simulink library "inp"  (R2021b)
settings: Solver=VariableStepAuto  StartTime=0.0  StopTime=10.0  RelTol=1e-3
undefined symbols (not defined in the file): C_TASK_5MS_S, FALSE, KINP_AcoreReadyToSlp_flg_ovrdflg, KINP_AcoreReadyToSlp_flg_ovrdval, KINP_AllowMovThd_OTA_enum_ovrdflg, KINP_AllowMovThd_OTA_enum_ovrdval, KINP_APSAngleTarget_Deg_ovrdflg, KINP_APSAngleTarget_Deg_ovrdval, KINP_APSDecReq_mps2_ovrdflg, KINP_APSDecReq_mps2_ovrdval, KINP_APSDecReqA_flg_ovrdflg, KINP_APSDecReqA_flg_ovrdval, KINP_APSDFLL_cm_ovrdflg, KINP_APSDFLL_cm_ovrdval, KINP_APSDFLR_cm_ovrdflg, KINP_APSDFLR_cm_ovrdval, KINP_APSDRLL_cm_ovrdflg, KINP_APSDRLL_cm_ovrdval, KINP_APSDRLR_cm_ovrdflg, KINP_APSDRLR_cm_ovrdval, KINP_APSExitCondition_enum_ovrdflg, KINP_APSExitCondition_enum_ovrdval, KINP_APSHWVer_enum_ovrdflg, KINP_APSHWVer_enum_ovrdval, KINP_APSProgressPCT_pct_ovrdflg, KINP_APSProgressPCT_pct_ovrdval, KINP_APSReq_enum_ovrdflg, KINP_APSReq_enum_ovrdval, KINP_APSRQDisplay_enum_ovrdflg, KINP_APSRQDisplay_enum_ovrdval, KINP_APSRqEPASCtrl_flg_ovrdflg, KINP_APSRqEPASCtrl_flg_ovrdval, KINP_APSShiftPosnReq_enum_ovrdval, KINP_APSShiftPosnReq_enum_ovrflg, KINP_APSSpeedCMD_kph_ovrdval, KINP_APSSpeedCMD_kph_ovrflg, KINP_APSStaSystem_enum_ovrdflg, KINP_APSStaSystem_enum_ovrdval, KINP_APSSWVer_enum_ovrdflg, KINP_APSSWVer_enum_ovrdval, KINP_APSVMCReqA_flg_ovrdval, KINP_APSVMCReqA_flg_ovrflg, KINP_APSVRqEPASCtrl_flg_ovrdflg, KINP_APSVRqEPASCtrl_flg_ovrdval, KINP_AuxBattVolmV_mV_ovrdflg, KINP_AuxBattVolmV_mV_ovrdval, KINP_CAASSta_enum_ovrdflg, KINP_CAASSta_enum_ovrdval, KINP_CAASVMCReqA_flg_ovrdval, KINP_CAASVMCReqA_flg_ovrflg, KINP_Chime_enum_ovrdflg, KINP_Chime_enum_ovrdval, KINP_ClearDTCcmd_flg_ovrdflg, KINP_ClearDTCcmd_flg_ovrdval, KINP_EvccAplusPwrUpReq_flg_ovrdflg, KINP_EvccAplusPwrUpReq_flg_ovrdval, KINP_LFID_raw_ovrdval, KINP_LFID_raw_ovrflg, KINP_LRID_raw_ovrdval, KINP_MemOffsetAccX_raw16_ovrdflg ... (+118)
libraries: FVT_lib x503, hcu_lib x1
(part 6 of 16)

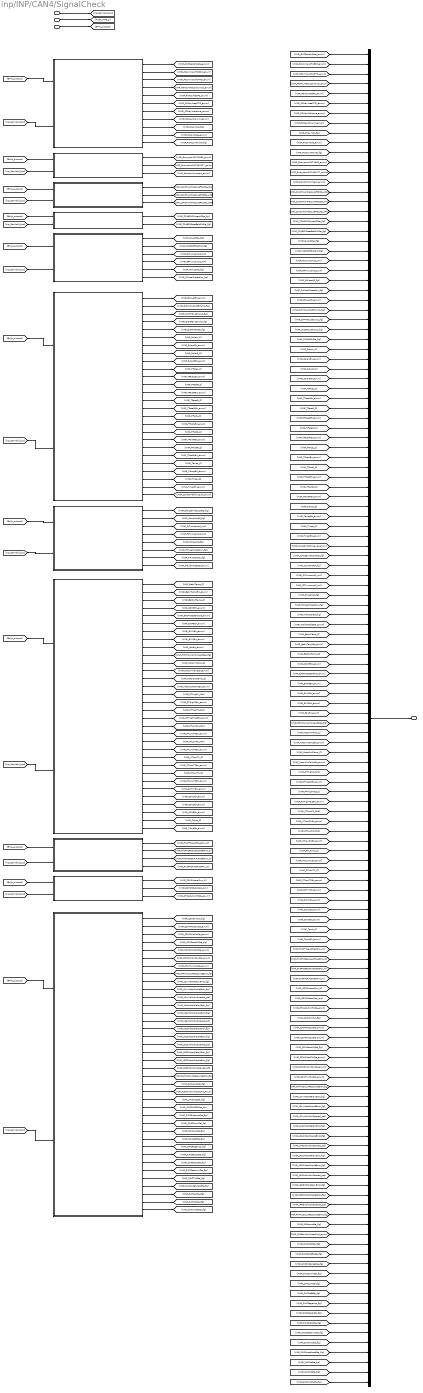
== system inp/INP/CAN4/SignalCheck ==
  inp_CanValid_bus : Inport
  TASK_TIME_S : Inport  Port=2
  BHAL_outputs : Inport  Port=3
  DKC1 : Subsystem
  DKC2 : Subsystem
  Z24_C1000_0 : Subsystem
  Z24_CE100_0 : Subsystem
  ZONE_DR1 : Subsystem
  ZONE_DR_VCU : Subsystem
  ZONE_FR1 : Subsystem
  ZONE_FR_VCU : Subsystem
  bus_creator : BusCreator  Inputs=136
  zGW_APTC1 : Subsystem
  zGW_CANFr1 : Subsystem
  zGW_LINDr1 : Subsystem
  inp_Hal_bus : Outport
  wires:
  inp_CanValid_bus/1 -> [inp_CanValid_bus]
  TASK_TIME_S/1 -> [TASK_TIME_S]
  BHAL_outputs/1 -> [BHAL_outputs]
  [BHAL_outputs] -> DKC1/1(BHAL_outputs)
  [inp_CanValid_bus] -> DKC1/2(inp_CanValid_bus)
  DKC1/1(VINP_DKCReVehData_enum) -> [VINP_DKCReVehData_enum]
  DKC1/2(VINP_PCommandToBCM_enum) -> [VINP_PCommandToBCM_enum]
  DKC1/3(VINP_PCommandToPTG_enum) -> [VINP_PCommandToPTG_enum]
  DKC1/4(VINP_PDKeyAreaLockUnlock_enum) -> [VINP_PDKeyAreaLockUnlock_enum]
  DKC1/5(VINP_PDKeyAreaPS_enum) -> [VINP_PDKeyAreaPS_enum]
  DKC1/6(VINP_PDKeyAreaPTG_enum) -> [VINP_PDKeyAreaPTG_enum]
  DKC1/7(VINP_PDKeyWelcome_enum) -> [VINP_PDKeyWelcome_enum]
  DKC1/8(VINP_PDkeyShowIVI_enum) -> [VINP_PDkeyShowIVI_enum]
  DKC1/9(VINP_PKeyMiss_flg) -> [VINP_PKeyMiss_flg]
  DKC1/10(VINP_PKeyMode_enum) -> [VINP_PKeyMode_enum]
  DKC1/11(VINP_PUIDLowPower_flg) -> [VINP_PUIDLowPower_flg]
  [BHAL_outputs] -> DKC2/1(BHAL_outputs)
  [inp_CanValid_bus] -> DKC2/2(inp_CanValid_bus)
  DKC2/1(VINP_EncryptionDATA063_enum) -> [VINP_EncryptionDATA063_enum]
  DKC2/2(VINP_EncryptionDATA64127_enum) -> [VINP_EncryptionDATA64127_enum]
  DKC2/3(VINP_RandomNumberX_enum) -> [VINP_RandomNumberX_enum]
  [BHAL_outputs] -> Z24_C1000_0/1(BHAL_outputs)
  [inp_CanValid_bus] -> Z24_C1000_0/2(inp_CanValid_bus)
  Z24_C1000_0/1(VINP_Z24CHAAirPressureFC2Sta_KPa) -> [VINP_Z24CHAAirPressureFC2Sta_KPa]
  Z24_C1000_0/2(VINP_Z24CHAAirPressurePC3Sta_KPa) -> [VINP_Z24CHAAirPressurePC3Sta_KPa]
  Z24_C1000_0/3(VINP_Z24CHAAirPressureRC1Sta_KPa) -> [VINP_Z24CHAAirPressureRC1Sta_KPa]
  [BHAL_outputs] -> Z24_CE100_0/1(BHAL_outputs)
  [inp_CanValid_bus] -> Z24_CE100_0/2(inp_CanValid_bus)
  Z24_CE100_0/1(VINP_Z24BCMFWiperASSta_flg) -> [VINP_Z24BCMFWiperASSta_flg]
  Z24_CE100_0/2(VINP_Z24BCMSeatBeltSWSta_flg) -> [VINP_Z24BCMSeatBeltSWSta_flg]
  [BHAL_outputs] -> ZONE_DR1/1(BHAL_outputs)
  [inp_CanValid_bus] -> ZONE_DR1/2(inp_CanValid_bus)
  ZONE_DR1/1(VINP_DrLockSta_flg) -> [VINP_DrLockSta_flg]
  ZONE_DR1/2(VINP_MIRRORFOLDSW_flg) -> [VINP_MIRRORFOLDSW_flg]
  ZONE_DR1/3(VINP_RLTurnLampC_mA) -> [VINP_RLTurnLampC_mA]
  ZONE_DR1/4(VINP_RRTurnLampC_mA) -> [VINP_RRTurnLampC_mA]
  ZONE_DR1/5(VINP_RWiperAS_flg) -> [VINP_RWiperAS_flg]
  ZONE_DR1/6(VINP_RWiperProtection_flg) -> [VINP_RWiperProtection_flg]
  [BHAL_outputs] -> ZONE_DR_VCU/1(BHAL_outputs)
  [inp_CanValid_bus] -> ZONE_DR_VCU/2(inp_CanValid_bus)
  ZONE_DR_VCU/1(VINP_BlowerErr_enum) -> [VINP_BlowerErr_enum]
  ZONE_DR_VCU/2(VINP_DrPMMLVOutPErrLmp_flg) -> [VINP_DrPMMLVOutPErrLmp_flg]
  ZONE_DR_VCU/3(VINP_DrPMMSysErrLmp_flg) -> [VINP_DrPMMSysErrLmp_flg]
  ZONE_DR_VCU/4(VINP_DrSCPSysErrLmp_flg) -> [VINP_DrSCPSysErrLmp_flg]
  ZONE_DR_VCU/5(VINP_DrStdAErrSta_flg) -> [VINP_DrStdAErrSta_flg]
  ZONE_DR_VCU/6(VINP_SolarL_W) -> [VINP_SolarL_W]
  ZONE_DR_VCU/7(VINP_SolarLErr_enum) -> [VINP_SolarLErr_enum]
  ZONE_DR_VCU/8(VINP_SolarR_W) -> [VINP_SolarR_W]
  ZONE_DR_VCU/9(VINP_SolarRErr_enum) -> [VINP_SolarRErr_enum]
  ZONE_DR_VCU/10(VINP_TFaceL_C) -> [VINP_TFaceL_C]
  ZONE_DR_VCU/11(VINP_TFaceLErr_enum) -> [VINP_TFaceLErr_enum]
  ZONE_DR_VCU/12(VINP_TFaceR_C) -> [VINP_TFaceR_C]
  ZONE_DR_VCU/13(VINP_TFaceRErr_enum) -> [VINP_TFaceRErr_enum]
  ZONE_DR_VCU/14(VINP_TFaceRr_C) -> [VINP_TFaceRr_C]
  ZONE_DR_VCU/15(VINP_TFaceRrErr_enum) -> [VINP_TFaceRrErr_enum]
  ZONE_DR_VCU/16(VINP_TFootL_C) -> [VINP_TFootL_C]
  ZONE_DR_VCU/17(VINP_TFootLErr_enum) -> [VINP_TFootLErr_enum]
  ZONE_DR_VCU/18(VINP_TFootR_C) -> [VINP_TFootR_C]
  ZONE_DR_VCU/19(VINP_TFootRErr_enum) -> [VINP_TFootRErr_enum]
  ZONE_DR_VCU/20(VINP_TFootRr_C) -> [VINP_TFootRr_C]
  ZONE_DR_VCU/21(VINP_TFootRrErr_enum) -> [VINP_TFootRrErr_enum]
  ZONE_DR_VCU/22(VINP_Tevap_C) -> [VINP_Tevap_C]
  ZONE_DR_VCU/23(VINP_TevapErr_enum) -> [VINP_TevapErr_enum]
  ZONE_DR_VCU/24(VINP_Tincar_C) -> [VINP_Tincar_C]
  ZONE_DR_VCU/25(VINP_TincarErr_enum) -> [VINP_TincarErr_enum]
  ZONE_DR_VCU/26(VINP_ZoneDrMalfunLevel_enum) -> [VINP_ZoneDrMalfunLevel_enum]
  [BHAL_outputs] -> ZONE_FR1/1(BHAL_outputs)
  [inp_CanValid_bus] -> ZONE_FR1/2(inp_CanValid_bus)
  ZONE_FR1/1(VINP_ChargeInletLockSta_flg) -> [VINP_ChargeInletLockSta_flg]
  ZONE_FR1/2(VINP_CompProEN_flg) -> [VINP_CompProEN_flg]
  ZONE_FR1/3(VINP_FLTurnLampC_mA) -> [VINP_FLTurnLampC_mA]
  ZONE_FR1/4(VINP_FRTurnLampC_mA) -> [VINP_FRTurnLampC_mA]
  ZONE_FR1/5(VINP_FWiperAS_flg) -> [VINP_FWiperAS_flg]
  ZONE_FR1/6(VINP_FWiperProtection_flg) -> [VINP_FWiperProtection_flg]
  ZONE_FR1/7(VINP_TrailerCheck_flg) -> [VINP_TrailerCheck_flg]
  ZONE_FR1/8(VINP_TrailerModeSta_enum) -> [VINP_TrailerModeSta_enum]
  [BHAL_outputs] -> ZONE_FR_VCU/1(BHAL_outputs)
  [inp_CanValid_bus] -> ZONE_FR_VCU/2(inp_CanValid_bus)
  ZONE_FR_VCU/1(VINP_BatInTemp_C) -> [VINP_BatInTemp_C]
  ZONE_FR_VCU/2(VINP_BatInTempErr_enum) -> [VINP_BatInTempErr_enum]
  ZONE_FR_VCU/3(VINP_BatOutTemp_C) -> [VINP_BatOutTemp_C]
  ZONE_FR_VCU/4(VINP_COMPErr_enum) -> [VINP_COMPErr_enum]
  ZONE_FR_VCU/5(VINP_EACProtectEnable_enum) -> [VINP_EACProtectEnable_enum]
  ZONE_FR_VCU/6(VINP_EWP3Err_enum) -> [VINP_EWP3Err_enum]
  ZONE_FR_VCU/7(VINP_EXV1Err_enum) -> [VINP_EXV1Err_enum]
  ZONE_FR_VCU/8(VINP_EXV2Err_enum) -> [VINP_EXV2Err_enum]
  ZONE_FR_VCU/9(VINP_FanErr_enum) -> [VINP_FanErr_enum]
  ZONE_FR_VCU/10(VINP_FrPMMLimpHomeActReq_flg) -> [VINP_FrPMMLimpHomeActReq_flg]
  ZONE_FR_VCU/11(VINP_MotorInTemp_C) -> [VINP_MotorInTemp_C]
  ZONE_FR_VCU/12(VINP_MotorInTempErr_enum) -> [VINP_MotorInTempErr_enum]
  ZONE_FR_VCU/13(VINP_MotorOutTemp_C) -> [VINP_MotorOutTemp_C]
  ZONE_FR_VCU/14(VINP_MotorOutTempErr_enum) -> [VINP_MotorOutTempErr_enum]
  ZONE_FR_VCU/15(VINP_PTHighP_KPa) -> [VINP_PTHighP_KPa]
  ZONE_FR_VCU/16(VINP_PTHighPErr_enum) -> [VINP_PTHighPErr_enum]
  ZONE_FR_VCU/17(VINP_PTHighTact_C) -> [VINP_PTHighTact_C]
  ZONE_FR_VCU/18(VINP_PTHighTactErr_enum) -> [VINP_PTHighTactErr_enum]
  ZONE_FR_VCU/19(VINP_PTLowP1_KPa) -> [VINP_PTLowP1_KPa]
  ZONE_FR_VCU/20(VINP_PTLowP1Err_enum) -> [VINP_PTLowP1Err_enum]
  ZONE_FR_VCU/21(VINP_PTLowP2_KPa) -> [VINP_PTLowP2_KPa]
  ZONE_FR_VCU/22(VINP_PTLowP2Err_enum) -> [VINP_PTLowP2Err_enum]
  ZONE_FR_VCU/23(VINP_PTLowT1_C) -> [VINP_PTLowT1_C]
  ZONE_FR_VCU/24(VINP_PTLowT1Err_enum) -> [VINP_PTLowT1Err_enum]
  ZONE_FR_VCU/25(VINP_PTLowT2_C) -> [VINP_PTLowT2_C]
  ZONE_FR_VCU/26(VINP_PTLowT2Err_enum) -> [VINP_PTLowT2Err_enum]
  ZONE_FR_VCU/27(VINP_SOTXVErr_enum) -> [VINP_SOTXVErr_enum]
  ZONE_FR_VCU/28(VINP_SOV1Err_enum) -> [VINP_SOV1Err_enum]
  ZONE_FR_VCU/29(VINP_SOV2Err_enum) -> [VINP_SOV2Err_enum]
  ZONE_FR_VCU/30(VINP_SOV3Err_enum) -> [VINP_SOV3Err_enum]
  ZONE_FR_VCU/31(VINP_Tamb_C) -> [VINP_Tamb_C]
  ZONE_FR_VCU/32(VINP_TambErr_enum) -> [VINP_TambErr_enum]
  [BHAL_outputs] -> zGW_APTC1/1(BHAL_outputs)
  [inp_CanValid_bus] -> zGW_APTC1/2(inp_CanValid_bus)
  zGW_APTC1/1(VINP_FrntPTCLeActHeatPwr_W) -> [VINP_FrntPTCLeActHeatPwr_W]
  zGW_APTC1/2(VINP_FrntPTCRearLeActHeatPwr_W) -> [VINP_FrntPTCRearLeActHeatPwr_W]
  zGW_APTC1/3(VINP_FrntPTCRearRiActHeatPwr_W) -> [VINP_FrntPTCRearRiActHeatPwr_W]
  zGW_APTC1/4(VINP_FrntPTCRiActHeatPwr_W) -> [VINP_FrntPTCRiActHeatPwr_W]
  [BHAL_outputs] -> zGW_CANFr1/1(BHAL_outputs)
  [inp_CanValid_bus] -> zGW_CANFr1/2(inp_CanValid_bus)
  zGW_CANFr1/1(VINP_COMPActualPwr_W) -> [VINP_COMPActualPwr_W]
  zGW_CANFr1/2(VINP_COMPStatorSpd_rpm) -> [VINP_COMPStatorSpd_rpm]
  zGW_CANFr1/3(VINP_PTCActuPwrHSC6_enum) -> [VINP_PTCActuPwrHSC6_enum]
  [BHAL_outputs] -> zGW_LINDr1/1(BHAL_outputs)
  [inp_CanValid_bus] -> zGW_LINDr1/2(inp_CanValid_bus)
  zGW_LINDr1/1(VINP_CSWDimSw_flg) -> [VINP_CSWDimSw_flg]
  zGW_LINDr1/2(VINP_CSWFWasSwSta_enum) -> [VINP_CSWFWasSwSta_enum]
  zGW_LINDr1/3(VINP_CSWFWipSwSta_enum) -> [VINP_CSWFWipSwSta_enum]
  zGW_LINDr1/4(VINP_CSWPassSWSta_flg) -> [VINP_CSWPassSWSta_flg]
  zGW_LINDr1/5(VINP_CSWRWasSWSta_enum) -> [VINP_CSWRWasSWSta_enum]
  zGW_LINDr1/6(VINP_CSWRWipIntSwSta_enum) -> [VINP_CSWRWipIntSwSta_enum]
  zGW_LINDr1/7(VINP_CSWTurnSwSta_enum) -> [VINP_CSWTurnSwSta_enum]
  zGW_LINDr1/8(VINP_FAPWL01LINResponseError_flg) -> [VINP_FAPWL01LINResponseError_flg]
  zGW_LINDr1/9(VINP_LDrvMotorRelayError_flg) -> [VINP_LDrvMotorRelayError_flg]
  zGW_LINDr1/10(VINP_LDrvMotorRippleError_flg) -> [VINP_LDrvMotorRippleError_flg]
  zGW_LINDr1/11(VINP_LDrvValWdwOpened_pct) -> [VINP_LDrvValWdwOpened_pct]
  zGW_LINDr1/12(VINP_LPasMotorRelayError_flg) -> [VINP_LPasMotorRelayError_flg]
  zGW_LINDr1/13(VINP_LPasMotorRippleError_flg) -> [VINP_LPasMotorRippleError_flg]
  zGW_LINDr1/14(VINP_LPasValWdwOpened_pct) -> [VINP_LPasValWdwOpened_pct]
  zGW_LINDr1/15(VINP_LRLDMotorRelayError_flg) -> [VINP_LRLDMotorRelayError_flg]
  zGW_LINDr1/16(VINP_LRLDMotorRippleError_flg) -> [VINP_LRLDMotorRippleError_flg]
  zGW_LINDr1/17(VINP_LRLDValWdwOpened_pct) -> [VINP_LRLDValWdwOpened_pct]
  zGW_LINDr1/18(VINP_LRRDMotorRelayError_flg) -> [VINP_LRRDMotorRelayError_flg]
  zGW_LINDr1/19(VINP_LRRDMotorRippleError_flg) -> [VINP_LRRDMotorRippleError_flg]
  zGW_LINDr1/20(VINP_LRRDValWdwOpened_pct) -> [VINP_LRRDValWdwOpened_pct]
  zGW_LINDr1/21(VINP_RAPWL01LINResponseError_flg) -> [VINP_RAPWL01LINResponseError_flg]
  zGW_LINDr1/22(VINP_RLSLampSta_flg) -> [VINP_RLSLampSta_flg]
  zGW_LINDr1/23(VINP_RLSRainSnrWiperCmd_enum) -> [VINP_RLSRainSnrWiperCmd_enum]
  zGW_LINDr1/24(VINP_SWCACCSta_flg) -> [VINP_SWCACCSta_flg]
  zGW_LINDr1/25(VINP_SWCCANCELSta_flg) -> [VINP_SWCCANCELSta_flg]
  zGW_LINDr1/26(VINP_SWCDistanceSta_flg) -> [VINP_SWCDistanceSta_flg]
  zGW_LINDr1/27(VINP_SWCDownSta_flg) -> [VINP_SWCDownSta_flg]
  zGW_LINDr1/28(VINP_SWCLKASta_flg) -> [VINP_SWCLKASta_flg]
  zGW_LINDr1/29(VINP_SWCLeftSta_flg) -> [VINP_SWCLeftSta_flg]
  zGW_LINDr1/30(VINP_SWCRegenUp_flg) -> [VINP_SWCRegenUp_flg]
  zGW_LINDr1/31(VINP_SWCResUpSta_flg) -> [VINP_SWCResUpSta_flg]
  zGW_LINDr1/32(VINP_SWCRightSta_flg) -> [VINP_SWCRightSta_flg]
  zGW_LINDr1/33(VINP_SWCSetdownSta_flg) -> [VINP_SWCSetdownSta_flg]
  zGW_LINDr1/34(VINP_SWCTripSta_flg) -> [VINP_SWCTripSta_flg]
  zGW_LINDr1/35(VINP_SWCUndefinedSta_flg) -> [VINP_SWCUndefinedSta_flg]
  zGW_LINDr1/36(VINP_SWCUpSta_flg) -> [VINP_SWCUpSta_flg]
  zGW_LINDr1/37(VINP_SWCVRSta_flg) -> [VINP_SWCVRSta_flg]
  zGW_LINDr1/38(VINP_SWCmodeSta_flg) -> [VINP_SWCmodeSta_flg]
  bus_creator/1 -> inp_Hal_bus/1
  [VINP_DKCReVehData_enum] -> bus_creator/1
  [VINP_PCommandToBCM_enum] -> bus_creator/2
  [VINP_PCommandToPTG_enum] -> bus_creator/3
  [VINP_PDKeyAreaLockUnlock_enum] -> bus_creator/4
  [VINP_PDKeyAreaPS_enum] -> bus_creator/5
  [VINP_PDKeyAreaPTG_enum] -> bus_creator/6
  [VINP_PDKeyWelcome_enum] -> bus_creator/7
  [VINP_PDkeyShowIVI_enum] -> bus_creator/8
  [VINP_PKeyMiss_flg] -> bus_creator/9
  [VINP_PKeyMode_enum] -> bus_creator/10
  [VINP_PUIDLowPower_flg] -> bus_creator/11
  [VINP_EncryptionDATA063_enum] -> bus_creator/12
  [VINP_EncryptionDATA64127_enum] -> bus_creator/13
  [VINP_RandomNumberX_enum] -> bus_creator/14
  [VINP_Z24CHAAirPressureFC2Sta_KPa] -> bus_creator/15
  [VINP_Z24CHAAirPressurePC3Sta_KPa] -> bus_creator/16
  [VINP_Z24CHAAirPressureRC1Sta_KPa] -> bus_creator/17
  [VINP_Z24BCMFWiperASSta_flg] -> bus_creator/18
  [VINP_Z24BCMSeatBeltSWSta_flg] -> bus_creator/19
  [VINP_DrLockSta_flg] -> bus_creator/20
  [VINP_MIRRORFOLDSW_flg] -> bus_creator/21
  [VINP_RLTurnLampC_mA] -> bus_creator/22
  [VINP_RRTurnLampC_mA] -> bus_creator/23
  [VINP_RWiperAS_flg] -> bus_creator/24
  [VINP_RWiperProtection_flg] -> bus_creator/25
  [VINP_BlowerErr_enum] -> bus_creator/26
  [VINP_DrPMMLVOutPErrLmp_flg] -> bus_creator/27
  [VINP_DrPMMSysErrLmp_flg] -> bus_creator/28
  [VINP_DrSCPSysErrLmp_flg] -> bus_creator/29
  [VINP_DrStdAErrSta_flg] -> bus_creator/30
  [VINP_SolarL_W] -> bus_creator/31
  [VINP_SolarLErr_enum] -> bus_creator/32
  [VINP_SolarR_W] -> bus_creator/33
  [VINP_SolarRErr_enum] -> bus_creator/34
  [VINP_TFaceL_C] -> bus_creator/35
  [VINP_TFaceLErr_enum] -> bus_creator/36
  [VINP_TFaceR_C] -> bus_creator/37
  [VINP_TFaceRErr_enum] -> bus_creator/38
  [VINP_TFaceRr_C] -> bus_creator/39
  [VINP_TFaceRrErr_enum] -> bus_creator/40
  [VINP_TFootL_C] -> bus_creator/41
  [VINP_TFootLErr_enum] -> bus_creator/42
  [VINP_TFootR_C] -> bus_creator/43
  [VINP_TFootRErr_enum] -> bus_creator/44
  [VINP_TFootRr_C] -> bus_creator/45
  [VINP_TFootRrErr_enum] -> bus_creator/46
  [VINP_Tevap_C] -> bus_creator/47
  [VINP_TevapErr_enum] -> bus_creator/48
  [VINP_Tincar_C] -> bus_creator/49
  [VINP_TincarErr_enum] -> bus_creator/50
  [VINP_ZoneDrMalfunLevel_enum] -> bus_creator/51
  [VINP_ChargeInletLockSta_flg] -> bus_creator/52
  [VINP_CompProEN_flg] -> bus_creator/53
  [VINP_FLTurnLampC_mA] -> bus_creator/54
  [VINP_FRTurnLampC_mA] -> bus_creator/55
  [VINP_FWiperAS_flg] -> bus_creator/56
  [VINP_FWiperProtection_flg] -> bus_creator/57
  [VINP_TrailerCheck_flg] -> bus_creator/58
  [VINP_TrailerModeSta_enum] -> bus_creator/59
  [VINP_BatInTemp_C] -> bus_creator/60
  [VINP_BatInTempErr_enum] -> bus_creator/61
  [VINP_BatOutTemp_C] -> bus_creator/62
  [VINP_COMPErr_enum] -> bus_creator/63
  [VINP_EACProtectEnable_enum] -> bus_creator/64
  [VINP_EWP3Err_enum] -> bus_creator/65
  [VINP_EXV1Err_enum] -> bus_creator/66
  [VINP_EXV2Err_enum] -> bus_creator/67
  [VINP_FanErr_enum] -> bus_creator/68
  [VINP_FrPMMLimpHomeActReq_flg] -> bus_creator/69
  [VINP_MotorInTemp_C] -> bus_creator/70
  [VINP_MotorInTempErr_enum] -> bus_creator/71
  [VINP_MotorOutTemp_C] -> bus_creator/72
  [VINP_MotorOutTempErr_enum] -> bus_creator/73
  [VINP_PTHighP_KPa] -> bus_creator/74
  [VINP_PTHighPErr_enum] -> bus_creator/75
  [VINP_PTHighTact_C] -> bus_creator/76
  [VINP_PTHighTactErr_enum] -> bus_creator/77
  [VINP_PTLowP1_KPa] -> bus_creator/78
  [VINP_PTLowP1Err_enum] -> bus_creator/79
  [VINP_PTLowP2_KPa] -> bus_creator/80
  [VINP_PTLowP2Err_enum] -> bus_creator/81
  [VINP_PTLowT1_C] -> bus_creator/82
  [VINP_PTLowT1Err_enum] -> bus_creator/83
  [VINP_PTLowT2_C] -> bus_creator/84
  [VINP_PTLowT2Err_enum] -> bus_creator/85
  [VINP_SOTXVErr_enum] -> bus_creator/86
  [VINP_SOV1Err_enum] -> bus_creator/87
  [VINP_SOV2Err_enum] -> bus_creator/88
  [VINP_SOV3Err_enum] -> bus_creator/89
  [VINP_Tamb_C] -> bus_creator/90
  [VINP_TambErr_enum] -> bus_creator/91
  [VINP_FrntPTCLeActHeatPwr_W] -> bus_creator/92
  [VINP_FrntPTCRearLeActHeatPwr_W] -> bus_creator/93
  [VINP_FrntPTCRearRiActHeatPwr_W] -> bus_creator/94
  [VINP_FrntPTCRiActHeatPwr_W] -> bus_creator/95
  [VINP_COMPActualPwr_W] -> bus_creator/96
  [VINP_COMPStatorSpd_rpm] -> bus_creator/97
  [VINP_PTCActuPwrHSC6_enum] -> bus_creator/98
  [VINP_CSWDimSw_flg] -> bus_creator/99
  [VINP_CSWFWasSwSta_enum] -> bus_creator/100
  [VINP_CSWFWipSwSta_enum] -> bus_creator/101
  [VINP_CSWPassSWSta_flg] -> bus_creator/102
  [VINP_CSWRWasSWSta_enum] -> bus_creator/103
  [VINP_CSWRWipIntSwSta_enum] -> bus_creator/104
  [VINP_CSWTurnSwSta_enum] -> bus_creator/105
  [VINP_FAPWL01LINResponseError_flg] -> bus_creator/106
  [VINP_LDrvMotorRelayError_flg] -> bus_creator/107
  [VINP_LDrvMotorRippleError_flg] -> bus_creator/108
  [VINP_LDrvValWdwOpened_pct] -> bus_creator/109
  [VINP_LPasMotorRelayError_flg] -> bus_creator/110
  [VINP_LPasMotorRippleError_flg] -> bus_creator/111
  [VINP_LPasValWdwOpened_pct] -> bus_creator/112
  [VINP_LRLDMotorRelayError_flg] -> bus_creator/113
  [VINP_LRLDMotorRippleError_flg] -> bus_creator/114
  [VINP_LRLDValWdwOpened_pct] -> bus_creator/115
  [VINP_LRRDMotorRelayError_flg] -> bus_creator/116
  [VINP_LRRDMotorRippleError_flg] -> bus_creator/117
  [VINP_LRRDValWdwOpened_pct] -> bus_creator/118
  [VINP_RAPWL01LINResponseError_flg] -> bus_creator/119
  [VINP_RLSLampSta_flg] -> bus_creator/120
  [VINP_RLSRainSnrWiperCmd_enum] -> bus_creator/121
  [VINP_SWCACCSta_flg] -> bus_creator/122
  [VINP_SWCCANCELSta_flg] -> bus_creator/123
  [VINP_SWCDistanceSta_flg] -> bus_creator/124
  [VINP_SWCDownSta_flg] -> bus_creator/125
  [VINP_SWCLKASta_flg] -> bus_creator/126
  [VINP_SWCLeftSta_flg] -> bus_creator/127
  [VINP_SWCRegenUp_flg] -> bus_creator/128
  [VINP_SWCResUpSta_flg] -> bus_creator/129
  [VINP_SWCRightSta_flg] -> bus_creator/130
  [VINP_SWCSetdownSta_flg] -> bus_creator/131
  [VINP_SWCTripSta_flg] -> bus_creator/132
  [VINP_SWCUndefinedSta_flg] -> bus_creator/133
  [VINP_SWCUpSta_flg] -> bus_creator/134
  [VINP_SWCVRSta_flg] -> bus_creator/135
  [VINP_SWCmodeSta_flg] -> bus_creator/136

== system inp/INP/CAN5/CommunicationCheck ==
  BHAL_outputs : Inport
  CANMsgInvalidTBOX1 : FVT_lib/inp/CAN_Msg_Validity_Process_template  SystemSampleTime=-1  VariantActivationTime=update diagram  Latency=0  AutoFrameSizeCalculation=off
      link override ovrdflg: Value=KINP_CANMsgInvalidTBOX1_flg_ovrdflg
      link override ovrdval: Value=KINP_CANMsgInvalidTBOX1_flg_ovrdval
  CANMsgInvalidTBOX2 : FVT_lib/inp/CAN_Msg_Validity_Process_template  SystemSampleTime=-1  VariantActivationTime=update diagram  Latency=0  AutoFrameSizeCalculation=off
      link override ovrdflg: Value=KINP_CANMsgInvalidTBOX2_flg_ovrdflg
      link override ovrdval: Value=KINP_CANMsgInvalidTBOX2_flg_ovrdval
  CANMsgInvalidTBOX3 : FVT_lib/inp/CAN_Msg_Validity_Process_template  SystemSampleTime=-1  VariantActivationTime=update diagram  Latency=0  AutoFrameSizeCalculation=off
      link override ovrdflg: Value=KINP_CANMsgInvalidTBOX3_flg_ovrdflg
      link override ovrdval: Value=KINP_CANMsgInvalidTBOX3_flg_ovrdval
  bus_creator : BusCreator  Inputs=3
  bus_selector : BusSelector  OutputSignals=VHAL_CANMsgInvalidTBOX1_flg,VHAL_CANMsgInvalidTBOX2_flg,VHAL_CANMsgInvalidTBOX3_flg
  not1 : Logic  Operator=NOT  AllPortsSameDT=off  OutDataTypeStr=boolean
  not2 : Logic  Operator=NOT  AllPortsSameDT=off  OutDataTypeStr=boolean
  not3 : Logic  Operator=NOT  AllPortsSameDT=off  OutDataTypeStr=boolean
  inp_CanValid_bus : Outport
  wires:
  BHAL_outputs/1 -> [BHAL_outputs]
  bus_selector/1 -> CANMsgInvalidTBOX1/1  "<VHAL_CANMsgInvalidTBOX1_flg>"
  CANMsgInvalidTBOX1/1 -> not1/1
  not1/1 -> bus_creator/1  "VINP_CANMsgValidTBOX1_flg"
  bus_selector/2 -> CANMsgInvalidTBOX2/1  "<VHAL_CANMsgInvalidTBOX2_flg>"
  CANMsgInvalidTBOX2/1 -> not2/1
  not2/1 -> bus_creator/2  "VINP_CANMsgValidTBOX2_flg"
  bus_selector/3 -> CANMsgInvalidTBOX3/1  "<VHAL_CANMsgInvalidTBOX3_flg>"
  CANMsgInvalidTBOX3/1 -> not3/1
  not3/1 -> bus_creator/3  "VINP_CANMsgValidTBOX3_flg"
  [BHAL_outputs] -> bus_selector/1
  bus_creator/1 -> inp_CanValid_bus/1

== system inp/INP/CAN5/CreateBus ==
  inp_CanValid_bus : Inport
  inp_Hal_bus : Inport  Port=2
  UnitConverter_{1..3,9,11} (5 alike) : DataTypeConversion  OutDataTypeStr=boolean
  UnitConverter_{5,10,14..30} (19 alike) : DataTypeConversion  OutDataTypeStr=single
  UnitConverter_{4,6,8,12..13} (5 alike) : DataTypeConversion  OutDataTypeStr=uint8
  UnitConverter_31 : DataTypeConversion  OutDataTypeStr=uint32
  UnitConverter_32 : DataTypeConversion  OutDataTypeStr=uint32
  UnitConverter_7 : DataTypeConversion  OutDataTypeStr=uint16
  bus_creator : BusCreator  Inputs=32
  bus_selector : BusSelector  OutputSignals=VINP_CANMsgValidTBOX1_flg,VINP_CANMsgValidTBOX2_flg,VINP_CANMsgValidTBOX3_flg
  bus_selector_1 : BusSelector  OutputSignals=VINP_CbnPreACEnaReq_enum,VINP_PowerOffTSet_cnt,VINP_ReOutsideMirror_enum,VINP_ReDoorLock_enum,VINP_RePwrReqTbox_enum,VINP_ReRadio_flg,VINP_RemoteACTemp_C,VINP_RemoteAutoReq_flg,VINP_TBOXNETSIGSTR_enum,VINP_TBOXTESTSTATUS_enum,VINP_TimeSyncFromBSDay_DAY,VINP_TimeSyncFromBSHour_hr,VINP_TimeSyncFromBSMinute_min,VINP_TimeSyncFromBSMonth_MONTH,VINP_TimeSyncFromBSSecond_s,VINP_TimeSyncFromBSYear_YEAR,VINP_ChargePercentSet_pct,VINP_ReserveChargeOFFDay_DAY,VINP_ReserveChargeOFFHour_hr,VINP_ReserveChargeOFFMinute_min,VINP_ReserveChargeOFFMonth_MONTH,VINP_ReserveChargeOFFYear_YEAR,VINP_ReserveChargeOnDay_DAY,VINP_ReserveChargeOnHour_hr,VINP_ReserveChargeOnMinute_min,VINP_ReserveChargeOnMonth_MONTH,VINP_ReserveChargeOnYear_YEAR,VINP_TBOXHWVER_enum,VINP_TBOXSWVER_enum
  BINP_outputs : Outport
  wires:
  inp_CanValid_bus/1 -> [inp_CanValid_bus]
  inp_Hal_bus/1 -> [inp_Hal_bus]
  bus_selector/1 -> UnitConverter_1/1  "<VINP_CANMsgValidTBOX1_flg>"
  UnitConverter_1/1 -> bus_creator/1  "VINP_CANMsgValidTBOX1_flg"
  bus_selector/2 -> UnitConverter_2/1  "<VINP_CANMsgValidTBOX2_flg>"
  UnitConverter_2/1 -> bus_creator/2  "VINP_CANMsgValidTBOX2_flg"
  bus_selector/3 -> UnitConverter_3/1  "<VINP_CANMsgValidTBOX3_flg>"
  UnitConverter_3/1 -> bus_creator/3  "VINP_CANMsgValidTBOX3_flg"
  bus_selector_1/1 -> UnitConverter_4/1  "<VINP_CbnPreACEnaReq_enum>"
  UnitConverter_4/1 -> bus_creator/4  "VINP_CbnPreACEnaReq_enum"
  bus_selector_1/2 -> UnitConverter_5/1  "<VINP_PowerOffTSet_cnt>"
  UnitConverter_5/1 -> bus_creator/5  "VINP_PowerOffTSet_cnt"
  bus_selector_1/3 -> UnitConverter_6/1  "<VINP_ReOutsideMirror_enum>"
  UnitConverter_6/1 -> bus_creator/6  "VINP_ReOutsideMirror_enum"
  bus_selector_1/4 -> UnitConverter_7/1  "<VINP_ReDoorLock_enum>"
  UnitConverter_7/1 -> bus_creator/7  "VINP_ReDoorLock_enum"
  bus_selector_1/5 -> UnitConverter_8/1  "<VINP_RePwrReqTbox_enum>"
  UnitConverter_8/1 -> bus_creator/8  "VINP_RePwrReqTbox_enum"
  bus_selector_1/6 -> UnitConverter_9/1  "<VINP_ReRadio_flg>"
  UnitConverter_9/1 -> bus_creator/9  "VINP_ReRadio_flg"
  bus_selector_1/7 -> UnitConverter_10/1  "<VINP_RemoteACTemp_C>"
  UnitConverter_10/1 -> bus_creator/10  "VINP_RemoteACTemp_C"
  bus_selector_1/8 -> UnitConverter_11/1  "<VINP_RemoteAutoReq_flg>"
  UnitConverter_11/1 -> bus_creator/11  "VINP_RemoteAutoReq_flg"
  bus_selector_1/9 -> UnitConverter_12/1  "<VINP_TBOXNETSIGSTR_enum>"
  UnitConverter_12/1 -> bus_creator/12  "VINP_TBOXNETSIGSTR_enum"
  bus_selector_1/10 -> UnitConverter_13/1  "<VINP_TBOXTESTSTATUS_enum>"
  UnitConverter_13/1 -> bus_creator/13  "VINP_TBOXTESTSTATUS_enum"
  bus_selector_1/11 -> UnitConverter_14/1  "<VINP_TimeSyncFromBSDay_DAY>"
  UnitConverter_14/1 -> bus_creator/14  "VINP_TimeSyncFromBSDay_DAY"
  bus_selector_1/12 -> UnitConverter_15/1  "<VINP_TimeSyncFromBSHour_hr>"
  UnitConverter_15/1 -> bus_creator/15  "VINP_TimeSyncFromBSHour_hr"
  bus_selector_1/13 -> UnitConverter_16/1  "<VINP_TimeSyncFromBSMinute_min>"
  UnitConverter_16/1 -> bus_creator/16  "VINP_TimeSyncFromBSMinute_min"
  bus_selector_1/14 -> UnitConverter_17/1  "<VINP_TimeSyncFromBSMonth_MONTH>"
  UnitConverter_17/1 -> bus_creator/17  "VINP_TimeSyncFromBSMonth_MONTH"
  bus_selector_1/15 -> UnitConverter_18/1  "<VINP_TimeSyncFromBSSecond_s>"
  UnitConverter_18/1 -> bus_creator/18  "VINP_TimeSyncFromBSSecond_s"
  bus_selector_1/16 -> UnitConverter_19/1  "<VINP_TimeSyncFromBSYear_YEAR>"
  UnitConverter_19/1 -> bus_creator/19  "VINP_TimeSyncFromBSYear_YEAR"
  bus_selector_1/17 -> UnitConverter_20/1  "<VINP_ChargePercentSet_pct>"
  UnitConverter_20/1 -> bus_creator/20  "VINP_ChargePercentSet_pct"
  bus_selector_1/18 -> UnitConverter_21/1  "<VINP_ReserveChargeOFFDay_DAY>"
  UnitConverter_21/1 -> bus_creator/21  "VINP_ReserveChargeOFFDay_DAY"
  bus_selector_1/19 -> UnitConverter_22/1  "<VINP_ReserveChargeOFFHour_hr>"
  UnitConverter_22/1 -> bus_creator/22  "VINP_ReserveChargeOFFHour_hr"
  bus_selector_1/20 -> UnitConverter_23/1  "<VINP_ReserveChargeOFFMinute_min>"
  UnitConverter_23/1 -> bus_creator/23  "VINP_ReserveChargeOFFMinute_min"
  bus_selector_1/21 -> UnitConverter_24/1  "<VINP_ReserveChargeOFFMonth_MONTH>"
  UnitConverter_24/1 -> bus_creator/24  "VINP_ReserveChargeOFFMonth_MONTH"
  bus_selector_1/22 -> UnitConverter_25/1  "<VINP_ReserveChargeOFFYear_YEAR>"
  UnitConverter_25/1 -> bus_creator/25  "VINP_ReserveChargeOFFYear_YEAR"
  bus_selector_1/23 -> UnitConverter_26/1  "<VINP_ReserveChargeOnDay_DAY>"
  UnitConverter_26/1 -> bus_creator/26  "VINP_ReserveChargeOnDay_DAY"
  bus_selector_1/24 -> UnitConverter_27/1  "<VINP_ReserveChargeOnHour_hr>"
  UnitConverter_27/1 -> bus_creator/27  "VINP_ReserveChargeOnHour_hr"
  bus_selector_1/25 -> UnitConverter_28/1  "<VINP_ReserveChargeOnMinute_min>"
  UnitConverter_28/1 -> bus_creator/28  "VINP_ReserveChargeOnMinute_min"
  bus_selector_1/26 -> UnitConverter_29/1  "<VINP_ReserveChargeOnMonth_MONTH>"
  UnitConverter_29/1 -> bus_creator/29  "VINP_ReserveChargeOnMonth_MONTH"
  bus_selector_1/27 -> UnitConverter_30/1  "<VINP_ReserveChargeOnYear_YEAR>"
  UnitConverter_30/1 -> bus_creator/30  "VINP_ReserveChargeOnYear_YEAR"
  bus_selector_1/28 -> UnitConverter_31/1  "<VINP_TBOXHWVER_enum>"
  UnitConverter_31/1 -> bus_creator/31  "VINP_TBOXHWVER_enum"
  bus_selector_1/29 -> UnitConverter_32/1  "<VINP_TBOXSWVER_enum>"
  UnitConverter_32/1 -> bus_creator/32  "VINP_TBOXSWVER_enum"
  [inp_CanValid_bus] -> bus_selector/1
  [inp_Hal_bus] -> bus_selector_1/1
  bus_creator/1 -> BINP_outputs/1

== system inp/INP/CAN5/SignalCheck ==
  inp_CanValid_bus : Inport
  TASK_TIME_S : Inport  Port=2
  BHAL_outputs : Inport  Port=3
  TBOX1 : Subsystem
  TBOX2 : Subsystem
  TBOX3 : Subsystem
  bus_creator : BusCreator  Inputs=29
  inp_Hal_bus : Outport
  wires:
  inp_CanValid_bus/1 -> [inp_CanValid_bus]
  TASK_TIME_S/1 -> [TASK_TIME_S]
  BHAL_outputs/1 -> [BHAL_outputs]
  [BHAL_outputs] -> TBOX1/1(BHAL_outputs)
  [inp_CanValid_bus] -> TBOX1/2(inp_CanValid_bus)
  TBOX1/1(VINP_CbnPreACEnaReq_enum) -> [VINP_CbnPreACEnaReq_enum]
  TBOX1/2(VINP_PowerOffTSet_cnt) -> [VINP_PowerOffTSet_cnt]
  TBOX1/3(VINP_ReOutsideMirror_enum) -> [VINP_ReOutsideMirror_enum]
  TBOX1/4(VINP_ReDoorLock_enum) -> [VINP_ReDoorLock_enum]
  TBOX1/5(VINP_RePwrReqTbox_enum) -> [VINP_RePwrReqTbox_enum]
  TBOX1/6(VINP_ReRadio_flg) -> [VINP_ReRadio_flg]
  TBOX1/7(VINP_RemoteACTemp_C) -> [VINP_RemoteACTemp_C]
  TBOX1/8(VINP_RemoteAutoReq_flg) -> [VINP_RemoteAutoReq_flg]
  TBOX1/9(VINP_TBOXNETSIGSTR_enum) -> [VINP_TBOXNETSIGSTR_enum]
  TBOX1/10(VINP_TBOXTESTSTATUS_enum) -> [VINP_TBOXTESTSTATUS_enum]
  [BHAL_outputs] -> TBOX2/1(BHAL_outputs)
  [inp_CanValid_bus] -> TBOX2/2(inp_CanValid_bus)
  TBOX2/1(VINP_TimeSyncFromBSDay_DAY) -> [VINP_TimeSyncFromBSDay_DAY]
  TBOX2/2(VINP_TimeSyncFromBSHour_hr) -> [VINP_TimeSyncFromBSHour_hr]
  TBOX2/3(VINP_TimeSyncFromBSMinute_min) -> [VINP_TimeSyncFromBSMinute_min]
  TBOX2/4(VINP_TimeSyncFromBSMonth_MONTH) -> [VINP_TimeSyncFromBSMonth_MONTH]
  TBOX2/5(VINP_TimeSyncFromBSSecond_s) -> [VINP_TimeSyncFromBSSecond_s]
  TBOX2/6(VINP_TimeSyncFromBSYear_YEAR) -> [VINP_TimeSyncFromBSYear_YEAR]
  [BHAL_outputs] -> TBOX3/1(BHAL_outputs)
  [inp_CanValid_bus] -> TBOX3/2(inp_CanValid_bus)
  TBOX3/1(VINP_ChargePercentSet_pct) -> [VINP_ChargePercentSet_pct]
  TBOX3/2(VINP_ReserveChargeOFFDay_DAY) -> [VINP_ReserveChargeOFFDay_DAY]
  TBOX3/3(VINP_ReserveChargeOFFHour_hr) -> [VINP_ReserveChargeOFFHour_hr]
  TBOX3/4(VINP_ReserveChargeOFFMinute_min) -> [VINP_ReserveChargeOFFMinute_min]
  TBOX3/5(VINP_ReserveChargeOFFMonth_MONTH) -> [VINP_ReserveChargeOFFMonth_MONTH]
  TBOX3/6(VINP_ReserveChargeOFFYear_YEAR) -> [VINP_ReserveChargeOFFYear_YEAR]
  TBOX3/7(VINP_ReserveChargeOnDay_DAY) -> [VINP_ReserveChargeOnDay_DAY]
  TBOX3/8(VINP_ReserveChargeOnHour_hr) -> [VINP_ReserveChargeOnHour_hr]
  TBOX3/9(VINP_ReserveChargeOnMinute_min) -> [VINP_ReserveChargeOnMinute_min]
  TBOX3/10(VINP_ReserveChargeOnMonth_MONTH) -> [VINP_ReserveChargeOnMonth_MONTH]
  TBOX3/11(VINP_ReserveChargeOnYear_YEAR) -> [VINP_ReserveChargeOnYear_YEAR]
  TBOX3/12(VINP_TBOXHWVER_enum) -> [VINP_TBOXHWVER_enum]
  TBOX3/13(VINP_TBOXSWVER_enum) -> [VINP_TBOXSWVER_enum]
  bus_creator/1 -> inp_Hal_bus/1
  [VINP_CbnPreACEnaReq_enum] -> bus_creator/1
  [VINP_PowerOffTSet_cnt] -> bus_creator/2
  [VINP_ReOutsideMirror_enum] -> bus_creator/3
  [VINP_ReDoorLock_enum] -> bus_creator/4
  [VINP_RePwrReqTbox_enum] -> bus_creator/5
  [VINP_ReRadio_flg] -> bus_creator/6
  [VINP_RemoteACTemp_C] -> bus_creator/7
  [VINP_RemoteAutoReq_flg] -> bus_creator/8
  [VINP_TBOXNETSIGSTR_enum] -> bus_creator/9
  [VINP_TBOXTESTSTATUS_enum] -> bus_creator/10
  [VINP_TimeSyncFromBSDay_DAY] -> bus_creator/11
  [VINP_TimeSyncFromBSHour_hr] -> bus_creator/12
  [VINP_TimeSyncFromBSMinute_min] -> bus_creator/13
  [VINP_TimeSyncFromBSMonth_MONTH] -> bus_creator/14
  [VINP_TimeSyncFromBSSecond_s] -> bus_creator/15
  [VINP_TimeSyncFromBSYear_YEAR] -> bus_creator/16
  [VINP_ChargePercentSet_pct] -> bus_creator/17
  [VINP_ReserveChargeOFFDay_DAY] -> bus_creator/18
  [VINP_ReserveChargeOFFHour_hr] -> bus_creator/19
  [VINP_ReserveChargeOFFMinute_min] -> bus_creator/20
  [VINP_ReserveChargeOFFMonth_MONTH] -> bus_creator/21
  [VINP_ReserveChargeOFFYear_YEAR] -> bus_creator/22
  [VINP_ReserveChargeOnDay_DAY] -> bus_creator/23
  [VINP_ReserveChargeOnHour_hr] -> bus_creator/24
  [VINP_ReserveChargeOnMinute_min] -> bus_creator/25
  [VINP_ReserveChargeOnMonth_MONTH] -> bus_creator/26
  [VINP_ReserveChargeOnYear_YEAR] -> bus_creator/27
  [VINP_TBOXHWVER_enum] -> bus_creator/28
  [VINP_TBOXSWVER_enum] -> bus_creator/29

== system inp/INP/CAN7/CommunicationCheck ==
  BHAL_outputs : Inport
  CANMsgInvalidDoorFr1 : FVT_lib/inp/CAN_Msg_Validity_Process_template  SystemSampleTime=-1  VariantActivationTime=update diagram  Latency=0  AutoFrameSizeCalculation=off
      link override ovrdflg: Value=KINP_CANMsgInvalidDoorFr1_flg_ovrdflg
      link override ovrdval: Value=KINP_CANMsgInvalidDoorFr1_flg_ovrdval
  bus_creator : BusCreator  Inputs=1
  bus_selector : BusSelector  OutputSignals=VHAL_CANMsgInvalidDoorFr1_flg
  not1 : Logic  Operator=NOT  AllPortsSameDT=off  OutDataTypeStr=boolean
  inp_CanValid_bus : Outport
  wires:
  BHAL_outputs/1 -> [BHAL_outputs]
  bus_selector/1 -> CANMsgInvalidDoorFr1/1  "<VHAL_CANMsgInvalidDoorFr1_flg>"
  CANMsgInvalidDoorFr1/1 -> not1/1
  not1/1 -> bus_creator/1  "VINP_CANMsgValidDoorFr1_flg"
  [BHAL_outputs] -> bus_selector/1
  bus_creator/1 -> inp_CanValid_bus/1

== system inp/INP/CAN7/CreateBus ==
  inp_CanValid_bus : Inport
  inp_Hal_bus : Inport  Port=2
  UnitConverter_1 : DataTypeConversion  OutDataTypeStr=boolean
  UnitConverter_2 : DataTypeConversion  OutDataTypeStr=uint8
  UnitConverter_3 : DataTypeConversion  OutDataTypeStr=uint8
  UnitConverter_4 : DataTypeConversion  OutDataTypeStr=uint8
  bus_creator : BusCreator  Inputs=4
  bus_selector : BusSelector  OutputSignals=VINP_CANMsgValidDoorFr1_flg
  bus_selector_1 : BusSelector  OutputSignals=VINP_DoorFrDoorEmergencysta_enum,VINP_DoorFrDooroperationsta_enum,VINP_DoorFrDoorpositionsta_enum
  BINP_outputs : Outport
  wires:
  inp_CanValid_bus/1 -> [inp_CanValid_bus]
  inp_Hal_bus/1 -> [inp_Hal_bus]
  bus_selector/1 -> UnitConverter_1/1  "<VINP_CANMsgValidDoorFr1_flg>"
  UnitConverter_1/1 -> bus_creator/1  "VINP_CANMsgValidDoorFr1_flg"
  bus_selector_1/1 -> UnitConverter_2/1  "<VINP_DoorFrDoorEmergencysta_enum>"
  UnitConverter_2/1 -> bus_creator/2  "VINP_DoorFrDoorEmergencysta_enum"
  bus_selector_1/2 -> UnitConverter_3/1  "<VINP_DoorFrDooroperationsta_enum>"
  UnitConverter_3/1 -> bus_creator/3  "VINP_DoorFrDooroperationsta_enum"
  bus_selector_1/3 -> UnitConverter_4/1  "<VINP_DoorFrDoorpositionsta_enum>"
  UnitConverter_4/1 -> bus_creator/4  "VINP_DoorFrDoorpositionsta_enum"
  [inp_CanValid_bus] -> bus_selector/1
  [inp_Hal_bus] -> bus_selector_1/1
  bus_creator/1 -> BINP_outputs/1

== system inp/INP/CAN7/SignalCheck ==
  inp_CanValid_bus : Inport
  TASK_TIME_S : Inport  Port=2
  BHAL_outputs : Inport  Port=3
  Door_Fr1 : Subsystem
  bus_creator : BusCreator  Inputs=3
  inp_Hal_bus : Outport
  wires:
  inp_CanValid_bus/1 -> [inp_CanValid_bus]
  TASK_TIME_S/1 -> [TASK_TIME_S]
  BHAL_outputs/1 -> [BHAL_outputs]
  [BHAL_outputs] -> Door_Fr1/1(BHAL_outputs)
  [inp_CanValid_bus] -> Door_Fr1/2(inp_CanValid_bus)
  Door_Fr1/1(VINP_DoorFrDoorEmergencysta_enum) -> [VINP_DoorFrDoorEmergencysta_enum]
  Door_Fr1/2(VINP_DoorFrDooroperationsta_enum) -> [VINP_DoorFrDooroperationsta_enum]
  Door_Fr1/3(VINP_DoorFrDoorpositionsta_enum) -> [VINP_DoorFrDoorpositionsta_enum]
  bus_creator/1 -> inp_Hal_bus/1
  [VINP_DoorFrDoorEmergencysta_enum] -> bus_creator/1
  [VINP_DoorFrDooroperationsta_enum] -> bus_creator/2
  [VINP_DoorFrDoorpositionsta_enum] -> bus_creator/3

== system inp/INP/GPIO/Analog ==
  BHAL_outputs : Inport
  TASK_TIME_S : Inport  Port=2
  AccelPedal1Vol_V : FVT_lib/inp/ad_signal_template  SystemSampleTime=-1  VariantActivationTime=update diagram  Latency=0  AutoFrameSizeCalculation=off
      link override defval: Value=KINP_AccelPedal1Vol_V_defval
      link override fftdec: Value=KINP_AccelPedal1Vol_V_fftdec
      link override fftinc: Value=KINP_AccelPedal1Vol_V_fftinc
      link override fftlim: Value=KINP_AccelPedal1Vol_V_fftlim
      link override limlow: Value=KINP_AccelPedal1Vol_V_limlow
      link override limupr: Value=KINP_AccelPedal1Vol_V_limupr
      link override ovrdflg: Value=KINP_AccelPedal1Vol_V_ovrdflg
      link override ovrdval: Value=KINP_AccelPedal1Vol_V_ovrdval
      link override srvcflg: Value=KINP_AccelPedal1Vol_V_srvcflg
      link override srvcval: Value=KINP_AccelPedal1Vol_V_srvcval
      link override tcfilt: Value=KINP_AccelPedal1Vol_V_tcfilt
  AccelPedal2Vol_V : FVT_lib/inp/ad_signal_template  SystemSampleTime=-1  VariantActivationTime=update diagram  Latency=0  AutoFrameSizeCalculation=off
      link override defval: Value=KINP_AccelPedal2Vol_V_defval
      link override fftdec: Value=KINP_AccelPedal2Vol_V_fftdec
      link override fftinc: Value=KINP_AccelPedal2Vol_V_fftinc
      link override fftlim: Value=KINP_AccelPedal2Vol_V_fftlim
      link override limlow: Value=KINP_AccelPedal2Vol_V_limlow
      link override limupr: Value=KINP_AccelPedal2Vol_V_limupr
      link override ovrdflg: Value=KINP_AccelPedal2Vol_V_ovrdflg
      link override ovrdval: Value=KINP_AccelPedal2Vol_V_ovrdval
      link override srvcflg: Value=KINP_AccelPedal2Vol_V_srvcflg
      link override srvcval: Value=KINP_AccelPedal2Vol_V_srvcval
      link override tcfilt: Value=KINP_AccelPedal2Vol_V_tcfilt
  Bus Selector : BusSelector  OutputSignals=VHAL_AccelPedal1Vol_V
  Bus Selector1 : BusSelector  OutputSignals=VHAL_AccelPedal2Vol_V
  Constant{,1..3} (4 alike) : Constant  Value=FALSE
  VINP_AccelPedal1VolShortHigh_enum : Outport
  VINP_AccelPedal1VolShortLow_enum : Outport  Port=2
  VINP_AccelPedal1Vol_V : Outport  Port=3
  VINP_AccelPedal1VolValid_flg : Outport  Port=4
  VINP_AccelPedal2VolShortHigh_enum : Outport  Port=5
  VINP_AccelPedal2VolShortLow_enum : Outport  Port=6
  VINP_AccelPedal2Vol_V : Outport  Port=7
  VINP_AccelPedal2VolValid_flg : Outport  Port=8
  wires:
  BHAL_outputs/1 -> [BHAL_outputs]
  TASK_TIME_S/1 -> [TASK_TIME_S]
  AccelPedal1Vol_V/1 -> VINP_AccelPedal1VolShortHigh_enum/1  "VINP_AccelPedal1VolShortHigh_enum"
  AccelPedal1Vol_V/2 -> VINP_AccelPedal1VolShortLow_enum/1  "VINP_AccelPedal1VolShortLow_enum"
  AccelPedal1Vol_V/3 -> VINP_AccelPedal1Vol_V/1  "VINP_AccelPedal1Vol_V"
  AccelPedal1Vol_V/4 -> VINP_AccelPedal1VolValid_flg/1  "VINP_AccelPedal1VolValid_flg"
  AccelPedal2Vol_V/1 -> VINP_AccelPedal2VolShortHigh_enum/1  "VINP_AccelPedal2VolShortHigh_enum"
  AccelPedal2Vol_V/2 -> VINP_AccelPedal2VolShortLow_enum/1  "VINP_AccelPedal2VolShortLow_enum"
  AccelPedal2Vol_V/3 -> VINP_AccelPedal2Vol_V/1  "VINP_AccelPedal2Vol_V"
  AccelPedal2Vol_V/4 -> VINP_AccelPedal2VolValid_flg/1  "VINP_AccelPedal2VolValid_flg"
  [TASK_TIME_S] -> AccelPedal1Vol_V/4
  Constant1/1 -> AccelPedal1Vol_V/3
  Constant/1 -> AccelPedal1Vol_V/2
  [BHAL_outputs] -> Bus Selector/1
  Bus Selector/1 -> AccelPedal1Vol_V/1  "<VHAL_AccelPedal1Vol_V>"
  Bus Selector1/1 -> AccelPedal2Vol_V/1  "<VHAL_AccelPedal2Vol_V>"
  [BHAL_outputs] -> Bus Selector1/1
  Constant2/1 -> AccelPedal2Vol_V/2
  Constant3/1 -> AccelPedal2Vol_V/3
  [TASK_TIME_S] -> AccelPedal2Vol_V/4

== system inp/INP/GPIO/Digital ==
  BHAL_outputs : Inport
  BrakeLampSW : FVT_lib/inp/di_signal_template  SystemSampleTime=-1  VariantActivationTime=update diagram  Latency=0  AutoFrameSizeCalculation=off
      link override debdec: Value=KINP_BrakeLampSW_flg_debdec
      link override debinc: Value=KINP_BrakeLampSW_flg_debinc
      link override deblim: Value=KINP_BrakeLampSW_flg_deblim
      link override inverse: Value=KINP_BrakeLampSW_flg_inverse
      link override ovrdflg: Value=KINP_BrakeLampSW_flg_ovrdflg
      link override ovrdval: Value=KINP_BrakeLampSW_flg_ovrdval
      link override srvcflg: Value=KINP_BrakeLampSW_flg_srvcflg
      link override srvcval: Value=KINP_BrakeLampSW_flg_srvcval
  BrakeSWGPIO : FVT_lib/inp/di_signal_template  SystemSampleTime=-1  VariantActivationTime=update diagram  Latency=0  AutoFrameSizeCalculation=off
      link override debdec: Value=KINP_BrakeSWGPIO_flg_debdec
      link override debinc: Value=KINP_BrakeSWGPIO_flg_debinc
      link override deblim: Value=KINP_BrakeSWGPIO_flg_deblim
      link override inverse: Value=KINP_BrakeSWGPIO_flg_inverse
      link override ovrdflg: Value=KINP_BrakeSWGPIO_flg_ovrdflg
      link override ovrdval: Value=KINP_BrakeSWGPIO_flg_ovrdval
      link override srvcflg: Value=KINP_BrakeSWGPIO_flg_srvcflg
      link override srvcval: Value=KINP_BrakeSWGPIO_flg_srvcval
  CentralDoorLockSW : FVT_lib/inp/di_signal_template  SystemSampleTime=-1  VariantActivationTime=update diagram  Latency=0  AutoFrameSizeCalculation=off
      link override debdec: Value=KINP_CentralDoorLockSW_flg_debdec
      link override debinc: Value=KINP_CentralDoorLockSW_flg_debinc
      link override deblim: Value=KINP_CentralDoorLockSW_flg_deblim
      link override inverse: Value=KINP_CentralDoorLockSW_flg_inverse
      link override ovrdflg: Value=KINP_CentralDoorLockSW_flg_ovrdflg
      link override ovrdval: Value=KINP_CentralDoorLockSW_flg_ovrdval
      link override srvcflg: Value=KINP_CentralDoorLockSW_flg_srvcflg
      link override srvcval: Value=KINP_CentralDoorLockSW_flg_srvcval
  CrashSignalGPIO : FVT_lib/inp/di_signal_template  SystemSampleTime=-1  VariantActivationTime=update diagram  Latency=0  AutoFrameSizeCalculation=off
      link override debdec: Value=KINP_CrashSignalGPIO_flg_debdec
      link override debinc: Value=KINP_CrashSignalGPIO_flg_debinc
      link override deblim: Value=KINP_CrashSignalGPIO_flg_deblim
      link override inverse: Value=KINP_CrashSignalGPIO_flg_inverse
      link override ovrdflg: Value=KINP_CrashSignalGPIO_flg_ovrdflg
      link override ovrdval: Value=KINP_CrashSignalGPIO_flg_ovrdval
      link override srvcflg: Value=KINP_CrashSignalGPIO_flg_srvcflg
      link override srvcval: Value=KINP_CrashSignalGPIO_flg_srvcval
  DrDoorSW : FVT_lib/inp/di_signal_template  SystemSampleTime=-1  VariantActivationTime=update diagram  Latency=0  AutoFrameSizeCalculation=off
      link override debdec: Value=KINP_DrDoorSW_flg_debdec
      link override debinc: Value=KINP_DrDoorSW_flg_debinc
      link override deblim: Value=KINP_DrDoorSW_flg_deblim
      link override inverse: Value=KINP_DrDoorSW_flg_inverse
      link override ovrdflg: Value=KINP_DrDoorSW_flg_ovrdflg
      link override ovrdval: Value=KINP_DrDoorSW_flg_ovrdval
      link override srvcflg: Value=KINP_DrDoorSW_flg_srvcflg
      link override srvcval: Value=KINP_DrDoorSW_flg_srvcval
  HazardSW : FVT_lib/inp/di_signal_template  SystemSampleTime=-1  VariantActivationTime=update diagram  Latency=0  AutoFrameSizeCalculation=off
      link override debdec: Value=KINP_HazardSW_flg_debdec
      link override debinc: Value=KINP_HazardSW_flg_debinc
      link override deblim: Value=KINP_HazardSW_flg_deblim
      link override inverse: Value=KINP_HazardSW_flg_inverse
      link override ovrdflg: Value=KINP_HazardSW_flg_ovrdflg
      link override ovrdval: Value=KINP_HazardSW_flg_ovrdval
      link override srvcflg: Value=KINP_HazardSW_flg_srvcflg
      link override srvcval: Value=KINP_HazardSW_flg_srvcval
  HoodSW : FVT_lib/inp/di_signal_template  SystemSampleTime=-1  VariantActivationTime=update diagram  Latency=0  AutoFrameSizeCalculation=off
      link override debdec: Value=KINP_HoodSW_flg_debdec
      link override debinc: Value=KINP_HoodSW_flg_debinc
      link override deblim: Value=KINP_HoodSW_flg_deblim
      link override inverse: Value=KINP_HoodSW_flg_inverse
      link override ovrdflg: Value=KINP_HoodSW_flg_ovrdflg
      link override ovrdval: Value=KINP_HoodSW_flg_ovrdval
      link override srvcflg: Value=KINP_HoodSW_flg_srvcflg
      link override srvcval: Value=KINP_HoodSW_flg_srvcval
  PsDoorSW : FVT_lib/inp/di_signal_template  SystemSampleTime=-1  VariantActivationTime=update diagram  Latency=0  AutoFrameSizeCalculation=off
      link override debdec: Value=KINP_PsDoorSW_flg_debdec
      link override debinc: Value=KINP_PsDoorSW_flg_debinc
      link override deblim: Value=KINP_PsDoorSW_flg_deblim
      link override inverse: Value=KINP_PsDoorSW_flg_inverse
      link override ovrdflg: Value=KINP_PsDoorSW_flg_ovrdflg
      link override ovrdval: Value=KINP_PsDoorSW_flg_ovrdval
      link override srvcflg: Value=KINP_PsDoorSW_flg_srvcflg
      link override srvcval: Value=KINP_PsDoorSW_flg_srvcval
  RLDoorSW : FVT_lib/inp/di_signal_template  SystemSampleTime=-1  VariantActivationTime=update diagram  Latency=0  AutoFrameSizeCalculation=off
      link override debdec: Value=KINP_RLDoorSW_flg_debdec
      link override debinc: Value=KINP_RLDoorSW_flg_debinc
      link override deblim: Value=KINP_RLDoorSW_flg_deblim
      link override inverse: Value=KINP_RLDoorSW_flg_inverse
      link override ovrdflg: Value=KINP_RLDoorSW_flg_ovrdflg
      link override ovrdval: Value=KINP_RLDoorSW_flg_ovrdval
      link override srvcflg: Value=KINP_RLDoorSW_flg_srvcflg
      link override srvcval: Value=KINP_RLDoorSW_flg_srvcval
  RRDoorSW : FVT_lib/inp/di_signal_template  SystemSampleTime=-1  VariantActivationTime=update diagram  Latency=0  AutoFrameSizeCalculation=off
      link override debdec: Value=KINP_RRDoorSW_flg_debdec
      link override debinc: Value=KINP_RRDoorSW_flg_debinc
      link override deblim: Value=KINP_RRDoorSW_flg_deblim
      link override inverse: Value=KINP_RRDoorSW_flg_inverse
      link override ovrdflg: Value=KINP_RRDoorSW_flg_ovrdflg
      link override ovrdval: Value=KINP_RRDoorSW_flg_ovrdval
      link override srvcflg: Value=KINP_RRDoorSW_flg_srvcflg
      link override srvcval: Value=KINP_RRDoorSW_flg_srvcval
  SeatSW : FVT_lib/inp/di_signal_template  SystemSampleTime=-1  VariantActivationTime=update diagram  Latency=0  AutoFrameSizeCalculation=off
      link override debdec: Value=KINP_SeatSW_flg_debdec
      link override debinc: Value=KINP_SeatSW_flg_debinc
      link override deblim: Value=KINP_SeatSW_flg_deblim
      link override inverse: Value=KINP_SeatSW_flg_inverse
      link override ovrdflg: Value=KINP_SeatSW_flg_ovrdflg
      link override ovrdval: Value=KINP_SeatSW_flg_ovrdval
      link override srvcflg: Value=KINP_SeatSW_flg_srvcflg
      link override srvcval: Value=KINP_SeatSW_flg_srvcval
  TailgateSW : FVT_lib/inp/di_signal_template  SystemSampleTime=-1  VariantActivationTime=update diagram  Latency=0  AutoFrameSizeCalculation=off
      link override debdec: Value=KINP_TailgateSW_flg_debdec
      link override debinc: Value=KINP_TailgateSW_flg_debinc
      link override deblim: Value=KINP_TailgateSW_flg_deblim
      link override inverse: Value=KINP_TailgateSW_flg_inverse
      link override ovrdflg: Value=KINP_TailgateSW_flg_ovrdflg
      link override ovrdval: Value=KINP_TailgateSW_flg_ovrdval
      link override srvcflg: Value=KINP_TailgateSW_flg_srvcflg
      link override srvcval: Value=KINP_TailgateSW_flg_srvcval
  TrunkHanSW : FVT_lib/inp/di_signal_template  SystemSampleTime=-1  VariantActivationTime=update diagram  Latency=0  AutoFrameSizeCalculation=off
      link override debdec: Value=KINP_TrunkHanSW_flg_debdec
      link override debinc: Value=KINP_TrunkHanSW_flg_debinc
      link override deblim: Value=KINP_TrunkHanSW_flg_deblim
      link override inverse: Value=KINP_TrunkHanSW_flg_inverse
      link override ovrdflg: Value=KINP_TrunkHanSW_flg_ovrdflg
      link override ovrdval: Value=KINP_TrunkHanSW_flg_ovrdval
      link override srvcflg: Value=KINP_TrunkHanSW_flg_srvcflg
      link override srvcval: Value=KINP_TrunkHanSW_flg_srvcval
  slr_VINP_BrakeLampSW_flg : BusSelector  OutputSignals=VHAL_BrakeLampSW_flg
  slr_VINP_BrakeSWGPIO_flg : BusSelector  OutputSignals=VHAL_BrakeSWGPIO_flg
  slr_VINP_CentralDoorLockSW_flg : BusSelector  OutputSignals=VHAL_CentralDoorLockSW_flg
  slr_VINP_CrashSignalGPIO_flg : BusSelector  OutputSignals=VHAL_CrashSignalGPIO_flg
  slr_VINP_DrDoorSW_flg : BusSelector  OutputSignals=VHAL_DrDoorSW_flg
  slr_VINP_HazardSW_flg : BusSelector  OutputSignals=VHAL_HazardSW_flg
  slr_VINP_HoodSW_flg : BusSelector  OutputSignals=VHAL_HoodSW_flg
  slr_VINP_PsDoorSW_flg : BusSelector  OutputSignals=VHAL_PsDoorSW_flg
  slr_VINP_RLDoorSW_flg : BusSelector  OutputSignals=VHAL_RLDoorSW_flg
  slr_VINP_RRDoorSW_flg : BusSelector  OutputSignals=VHAL_RRDoorSW_flg
  slr_VINP_SeatSW_flg : BusSelector  OutputSignals=VHAL_SeatSW_flg
  slr_VINP_TailgateSW_flg : BusSelector  OutputSignals=VHAL_TailgateSW_flg
  slr_VINP_TrunkHanSW_flg : BusSelector  OutputSignals=VHAL_TrunkHanSW_flg
  VINP_BrakeSWGPIO_flg : Outport
  VINP_HoodSW_flg : Outport  Port=2
  VINP_TailgateSW_flg : Outport  Port=3
  VINP_DrDoorSW_flg : Outport  Port=4
  VINP_PsDoorSW_flg : Outport  Port=5
  VINP_RRDoorSW_flg : Outport  Port=6
  VINP_RLDoorSW_flg : Outport  Port=7
  VINP_CentralDoorLockSW_flg : Outport  Port=8
  VINP_HazardSW_flg : Outport  Port=9
  VINP_BrakeLampSW_flg : Outport  Port=10
  VINP_TrunkHanSW_flg : Outport  Port=11
  VINP_SeatSW_flg : Outport  Port=12
  VINP_CrashSignalGPIO_flg : Outport  Port=13
  wires:
  BHAL_outputs/1 -> [BHAL_outputs]
  BrakeSWGPIO/1 -> VINP_BrakeSWGPIO_flg/1  "VINP_BrakeSWGPIO_flg"
  [BHAL_outputs] -> slr_VINP_BrakeSWGPIO_flg/1
  slr_VINP_BrakeSWGPIO_flg/1 -> BrakeSWGPIO/1  "<VHAL_BrakeSWGPIO_flg>"
  HoodSW/1 -> VINP_HoodSW_flg/1  "VINP_HoodSW_flg"
  [BHAL_outputs] -> slr_VINP_HoodSW_flg/1
  slr_VINP_HoodSW_flg/1 -> HoodSW/1  "<VHAL_HoodSW_flg>"
  TailgateSW/1 -> VINP_TailgateSW_flg/1  "VINP_TailgateSW_flg"
  [BHAL_outputs] -> slr_VINP_TailgateSW_flg/1
  slr_VINP_TailgateSW_flg/1 -> TailgateSW/1  "<VHAL_TailgateSW_flg>"
  DrDoorSW/1 -> VINP_DrDoorSW_flg/1  "VINP_DrDoorSW_flg"
  [BHAL_outputs] -> slr_VINP_DrDoorSW_flg/1
  slr_VINP_DrDoorSW_flg/1 -> DrDoorSW/1  "<VHAL_DrDoorSW_flg>"
  PsDoorSW/1 -> VINP_PsDoorSW_flg/1  "VINP_PsDoorSW_flg"
  [BHAL_outputs] -> slr_VINP_PsDoorSW_flg/1
  slr_VINP_PsDoorSW_flg/1 -> PsDoorSW/1  "<VHAL_PsDoorSW_flg>"
  RRDoorSW/1 -> VINP_RRDoorSW_flg/1  "VINP_RRDoorSW_flg"
  [BHAL_outputs] -> slr_VINP_RRDoorSW_flg/1
  slr_VINP_RRDoorSW_flg/1 -> RRDoorSW/1  "<VHAL_RRDoorSW_flg>"
  RLDoorSW/1 -> VINP_RLDoorSW_flg/1  "VINP_RLDoorSW_flg"
  [BHAL_outputs] -> slr_VINP_RLDoorSW_flg/1
  slr_VINP_RLDoorSW_flg/1 -> RLDoorSW/1  "<VHAL_RLDoorSW_flg>"
  CentralDoorLockSW/1 -> VINP_CentralDoorLockSW_flg/1  "VINP_CentralDoorLockSW_flg"
  [BHAL_outputs] -> slr_VINP_CentralDoorLockSW_flg/1
  slr_VINP_CentralDoorLockSW_flg/1 -> CentralDoorLockSW/1  "<VHAL_CentralDoorLockSW_flg>"
  HazardSW/1 -> VINP_HazardSW_flg/1  "VINP_HazardSW_flg"
  [BHAL_outputs] -> slr_VINP_HazardSW_flg/1
  slr_VINP_HazardSW_flg/1 -> HazardSW/1  "<VHAL_HazardSW_flg>"
  BrakeLampSW/1 -> VINP_BrakeLampSW_flg/1  "VINP_BrakeLampSW_flg"
  [BHAL_outputs] -> slr_VINP_BrakeLampSW_flg/1
  slr_VINP_BrakeLampSW_flg/1 -> BrakeLampSW/1  "<VHAL_BrakeLampSW_flg>"
  TrunkHanSW/1 -> VINP_TrunkHanSW_flg/1  "VINP_TrunkHanSW_flg"
  [BHAL_outputs] -> slr_VINP_TrunkHanSW_flg/1
  slr_VINP_TrunkHanSW_flg/1 -> TrunkHanSW/1  "<VHAL_TrunkHanSW_flg>"
  SeatSW/1 -> VINP_SeatSW_flg/1  "VINP_SeatSW_flg"
  [BHAL_outputs] -> slr_VINP_SeatSW_flg/1
  slr_VINP_SeatSW_flg/1 -> SeatSW/1  "<VHAL_SeatSW_flg>"
  [BHAL_outputs] -> slr_VINP_CrashSignalGPIO_flg/1
  slr_VINP_CrashSignalGPIO_flg/1 -> CrashSignalGPIO/1  "<VHAL_CrashSignalGPIO_flg>"
  CrashSignalGPIO/1 -> VINP_CrashSignalGPIO_flg/1  "VINP_CrashSignalGPIO_flg"

== system inp/INP/IMU/Subsystem1 ==
  In1 : Inport
  Constant : Constant  Value=KINP_MemOffsetGyroY_raw16_ovrdval
  Constant1 : Constant  Value=KINP_MemOffsetGyroY_raw16_ovrdflg
  Switch : Switch  Criteria=u2 ~= 0
  Out1 : Outport
  wires:
  Switch/1 -> Out1/1
  Constant/1 -> Switch/1
  Constant1/1 -> Switch/2
  In1/1 -> Switch/3
